simulink model "P_n_2015a"  (R2015a)
settings: Solver=ode45  StartTime=0.0  StopTime=100  RelTol=1e-3
undefined symbols (not defined in the file or in its folder): C, phi
settings Model: CovModelRefEnable=off  Creator=lucasperovani  LastModifiedBy=lucasperovani
settings DataIOCC: SaveFormat=Dataset
settings HardwareCC: ProdBitPerPointer=64  ProdLargestAtomicFloat=Float  ProdIntDivRoundTo=Zero  ProdEndianess=LittleEndian  ProdHWDeviceType=Specified
settings GRTTargetCC: GeneratePreprocessorConditionals=Use local settings

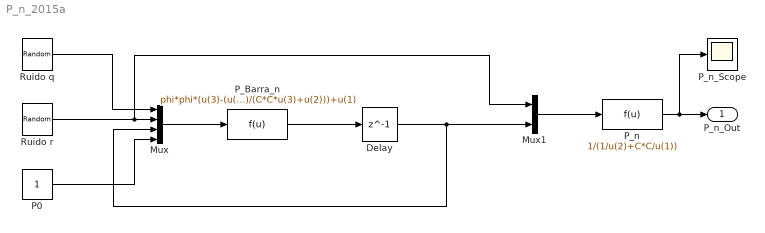
== system P_n_2015a ==
  Delay : Delay  DelayLength=1  InitialCondition=0
  Mux : Mux
  Mux1 : Mux  Inputs=2
  P0 : Constant  SampleTime=1
  P_Barra_n : Fcn  Expr=phi*phi*(u(3)-(u(3)*u(3)*C*C)/(C*C*u(3)+u(2)))+u(1)
  P_n : Fcn  Expr=1/(1/u(2)+C*C/u(1))
  "P_n_Scope " : Scope
      settings: TimeRange=auto  MaxDataPoints=5000  SaveToWorkspace=off  SaveName=ScopeData  YMin=-606.22567  YMax=675.8399  SampleTime=-1
  Ruido q : UniformRandomNumber  SampleTime=0.1
  Ruido r : UniformRandomNumber  SampleTime=0.1
  P_n_Out : Outport
  wires:
  P_Barra_n/1 -> Delay/1
  Mux/1 -> P_Barra_n/1
  Delay/1 -> Mux1/2, Mux/3
  Ruido r/1 -> Mux1/1, Mux/2
  Ruido q/1 -> Mux/1
  Mux1/1 -> P_n/1
  P_n/1 -> "P_n_Scope "/1, P_n_Out/1
  P0/1 -> Mux/4
